simulink model "PD_controller_plant"  (R2024b)
settings: Solver=FixedStepAuto  StartTime=0.0  StopTime=120  FixedStep=0.0001  RelTol=1e-3
values from neighbouring files (symbols this model uses):
  A = [-d1 0 1; 0 0 1; d3 0 d4]    [PDD_Sweep.m]    (also in PD_Controller.m)
  B = [-d5; 0; d2]    [PDD_Sweep.m]    (also in PD_Controller.m)
  C = eye(3)    [PD_Controller.m]
  D = [0; 0; 0]    [PD_Controller.m]
  K = [K_alpha, 0, K_q]    [PD_Controller.m]
  x0 = [2*pi/180; 0; 0;]    [PD_Controller.m]
libraries: simulink_extras x3, aerolibactuator x1
settings Model: Creator=jonno  LastModifiedBy=jonno

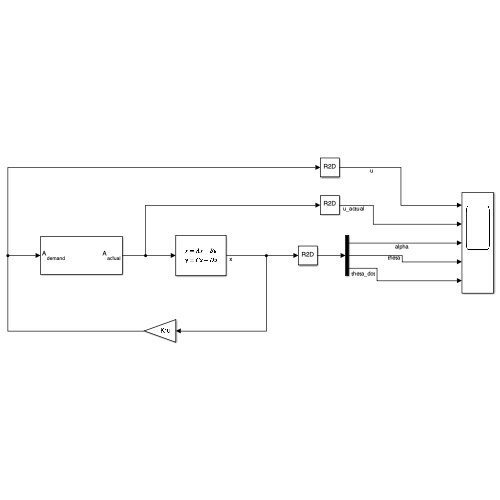
[thumbnail: Simulink's stored preview of the top-level diagram]
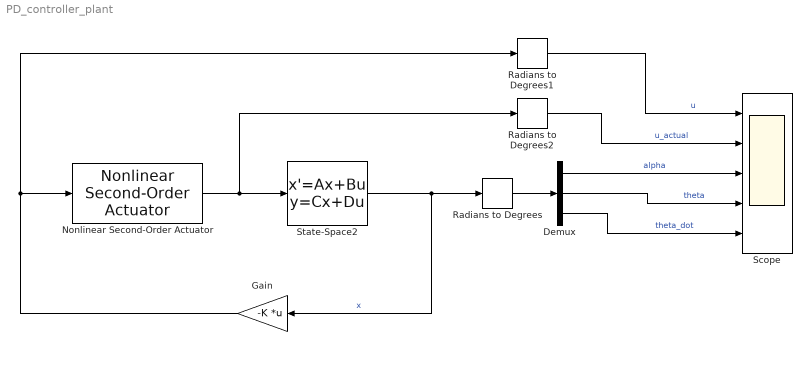
== system PD_controller_plant ==
  Demux : Demux  Outputs=3
  Gain : Gain  Gain=-K  Multiplication=Matrix(K*u)
  Nonlinear Second-Order Actuator : aerolibactuator/Nonlinear Second-Order Actuator  wn_fin=65  z_fin=0.7  fin_max=20*pi/180  fin_min=-20*pi/180  fin_maxrate=500*pi/180  fin_act_0=0  fin_act_vel=0
  Radians to Degrees : simulink_extras/Transformations/Radians to Degrees
  Radians to Degrees1 : simulink_extras/Transformations/Radians to Degrees
  Radians to Degrees2 : simulink_extras/Transformations/Radians to Degrees
  Scope : Scope  NumInputPorts=5
  State-Space2 : StateSpace  A=A  B=B  C=C  D=D  InitialCondition=x0
  wires:
  State-Space2/1 -> Gain/1, Radians to Degrees/1  "x"
  Radians to Degrees/1 -> Demux/1
  Demux/1 -> Scope/3  "alpha"
  Demux/2 -> Scope/4  "theta"
  Demux/3 -> Scope/5  "theta_dot"
  Gain/1 -> Nonlinear Second-Order Actuator/1, Radians to Degrees1/1
  Radians to Degrees1/1 -> Scope/1  "u"
  Nonlinear Second-Order Actuator/1 -> Radians to Degrees2/1, State-Space2/1
  Radians to Degrees2/1 -> Scope/2  "u_actual"
